simulink model "VAS_LEVEL0_TASK1_TIME"  (Simulink 3.00)
libraries: mathlib x438, logiclib x192, paramlib x18, genlib x3, timelib x1
(part 2 of 2)

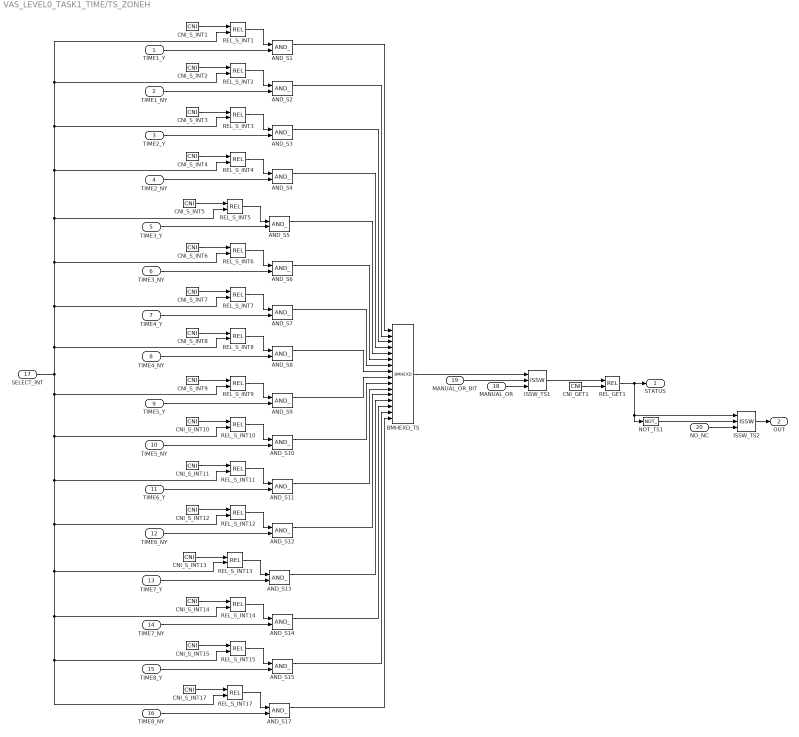
== system VAS_LEVEL0_TASK1_TIME/TS_ZONEH ==
  TIME1_Y : Inport  Port=1
  TIME1_NY : Inport  Port=2
  TIME2_Y : Inport  Port=3
  TIME2_NY : Inport  Port=4
  TIME3_Y : Inport  Port=5
  TIME3_NY : Inport  Port=6
  TIME4_Y : Inport  Port=7
  TIME4_NY : Inport  Port=8
  TIME5_Y : Inport  Port=9
  TIME5_NY : Inport  Port=10
  TIME6_Y : Inport  Port=11
  TIME6_NY : Inport  Port=12
  TIME7_Y : Inport  Port=13
  TIME7_NY : Inport  Port=14
  TIME8_Y : Inport  Port=15
  TIME8_NY : Inport  Port=16
  SELECT_INT : Inport  Port=17
  MANUAL_OR : Inport  Port=18
  MANUAL_OR_BIT : Inport  Port=19
  NO_NC : Inport  Port=20
  AND_S{1..15,17} (16 alike) : logiclib/AND_
  BMHEXD_TS : logiclib/BMHEXD  shift=0
  CNI_GET1 : mathlib/CNI  icn=1
  CNI_S_INT1 : mathlib/CNI  icn=0
  CNI_S_INT10 : mathlib/CNI  icn=9
  CNI_S_INT11 : mathlib/CNI  icn=10
  CNI_S_INT12 : mathlib/CNI  icn=11
  CNI_S_INT13 : mathlib/CNI  icn=12
  CNI_S_INT14 : mathlib/CNI  icn=13
  CNI_S_INT15 : mathlib/CNI  icn=14
  CNI_S_INT17 : mathlib/CNI  icn=15
  CNI_S_INT2 : mathlib/CNI  icn=1
  CNI_S_INT3 : mathlib/CNI  icn=2
  CNI_S_INT4 : mathlib/CNI  icn=3
  CNI_S_INT5 : mathlib/CNI  icn=4
  CNI_S_INT6 : mathlib/CNI  icn=5
  CNI_S_INT7 : mathlib/CNI  icn=6
  CNI_S_INT8 : mathlib/CNI  icn=7
  CNI_S_INT9 : mathlib/CNI  icn=8
  ISSW_TS1 : logiclib/ISSW
  ISSW_TS2 : logiclib/ISSW
  NOT_TS1 : logiclib/NOT_
  REL_GET1 : mathlib/REL  irel=6: greater or equal (>=)
  REL_S_INT{1..15,17} (16 alike) : mathlib/REL  irel=1: equality (==)
  STATUS : Outport  Port=1
  OUT : Outport  Port=2
  wires:
  AND_S1/1 -> BMHEXD_TS/1
  AND_S10/1 -> BMHEXD_TS/10
  AND_S11/1 -> BMHEXD_TS/11
  AND_S12/1 -> BMHEXD_TS/12
  AND_S13/1 -> BMHEXD_TS/13
  AND_S14/1 -> BMHEXD_TS/14
  AND_S15/1 -> BMHEXD_TS/15
  AND_S17/1 -> BMHEXD_TS/16
  AND_S2/1 -> BMHEXD_TS/2
  AND_S3/1 -> BMHEXD_TS/3
  AND_S4/1 -> BMHEXD_TS/4
  AND_S5/1 -> BMHEXD_TS/5
  AND_S6/1 -> BMHEXD_TS/6
  AND_S7/1 -> BMHEXD_TS/7
  AND_S8/1 -> BMHEXD_TS/8
  AND_S9/1 -> BMHEXD_TS/9
  BMHEXD_TS/1 -> ISSW_TS1/1
  CNI_GET1/1 -> REL_GET1/2
  CNI_S_INT1/1 -> REL_S_INT1/1
  CNI_S_INT10/1 -> REL_S_INT10/1
  CNI_S_INT11/1 -> REL_S_INT11/1
  CNI_S_INT12/1 -> REL_S_INT12/1
  CNI_S_INT13/1 -> REL_S_INT13/1
  CNI_S_INT14/1 -> REL_S_INT14/1
  CNI_S_INT15/1 -> REL_S_INT15/1
  CNI_S_INT17/1 -> REL_S_INT17/1
  CNI_S_INT2/1 -> REL_S_INT2/1
  CNI_S_INT3/1 -> REL_S_INT3/1
  CNI_S_INT4/1 -> REL_S_INT4/1
  CNI_S_INT5/1 -> REL_S_INT5/1
  CNI_S_INT6/1 -> REL_S_INT6/1
  CNI_S_INT7/1 -> REL_S_INT7/1
  CNI_S_INT8/1 -> REL_S_INT8/1
  CNI_S_INT9/1 -> REL_S_INT9/1
  ISSW_TS1/1 -> REL_GET1/1
  ISSW_TS2/1 -> OUT/1
  MANUAL_OR/1 -> ISSW_TS1/3
  MANUAL_OR_BIT/1 -> ISSW_TS1/2
  NOT_TS1/1 -> ISSW_TS2/2
  NO_NC/1 -> ISSW_TS2/3
  REL_GET1/1 -> STATUS/1, ISSW_TS2/1, NOT_TS1/1
  REL_S_INT1/1 -> AND_S1/1
  REL_S_INT10/1 -> AND_S10/1
  REL_S_INT11/1 -> AND_S11/1
  REL_S_INT12/1 -> AND_S12/1
  REL_S_INT13/1 -> AND_S13/1
  REL_S_INT14/1 -> AND_S14/1
  REL_S_INT15/1 -> AND_S15/1
  REL_S_INT17/1 -> AND_S17/1
  REL_S_INT2/1 -> AND_S2/1
  REL_S_INT3/1 -> AND_S3/1
  REL_S_INT4/1 -> AND_S4/1
  REL_S_INT5/1 -> AND_S5/1
  REL_S_INT6/1 -> AND_S6/1
  REL_S_INT7/1 -> AND_S7/1
  REL_S_INT8/1 -> AND_S8/1
  REL_S_INT9/1 -> AND_S9/1
  SELECT_INT/1 -> REL_S_INT1/2, REL_S_INT2/2, REL_S_INT3/2, REL_S_INT4/2, REL_S_INT5/2, REL_S_INT6/2, REL_S_INT7/2, REL_S_INT8/2, REL_S_INT14/2, REL_S_INT15/2, REL_S_INT17/2, REL_S_INT13/2, REL_S_INT12/2, REL_S_INT11/2, REL_S_INT10/2, REL_S_INT9/2
  TIME1_NY/1 -> AND_S2/2
  TIME1_Y/1 -> AND_S1/2
  TIME2_NY/1 -> AND_S4/2
  TIME2_Y/1 -> AND_S3/2
  TIME3_NY/1 -> AND_S6/2
  TIME3_Y/1 -> AND_S5/2
  TIME4_NY/1 -> AND_S8/2
  TIME4_Y/1 -> AND_S7/2
  TIME5_NY/1 -> AND_S10/2
  TIME5_Y/1 -> AND_S9/2
  TIME6_NY/1 -> AND_S12/2
  TIME6_Y/1 -> AND_S11/2
  TIME7_NY/1 -> AND_S14/2
  TIME7_Y/1 -> AND_S13/2
  TIME8_NY/1 -> AND_S17/2
  TIME8_Y/1 -> AND_S15/2

== system VAS_LEVEL0_TASK1_TIME/EPHEM_CTBE/EPHEM_BEGIN ==
  ENABLE : Inport  Port=1
  ADD_AMS : mathlib/ADD
  ADD_HM : mathlib/ADD
  CNI_IMUL_H : mathlib/CNI  icn=3600
  CNI_IMUL_M : mathlib/CNI  icn=60
  MUL_H : mathlib/MUL
  MUL_M : mathlib/MUL
  SILO_HOUR : paramlib/SILO  fname=/ramdisk/begin_civil_twilight/loc_hour.txt  CSF=off  CLF=off  yerr=0
  SILO_MINUTE : paramlib/SILO  fname=/ramdisk/begin_civil_twilight/loc_minute.txt  CSF=off  CLF=off  yerr=0
  SILO_SECONDS : paramlib/SILO  fname=/ramdisk/begin_civil_twilight/loc_secound.txt  CSF=off  CLF=off  yerr=0
  HOUR : Outport  Port=1
  MINUTE : Outport  Port=2
  SECONDS : Outport  Port=3
  SEC_OF_DAY : Outport  Port=4
  wires:
  ADD_AMS/1 -> SEC_OF_DAY/1
  ADD_HM/1 -> ADD_AMS/1
  CNI_IMUL_H/1 -> MUL_H/2
  CNI_IMUL_M/1 -> MUL_M/2
  ENABLE/1 -> SILO_HOUR/3, SILO_MINUTE/3, SILO_SECONDS/3
  MUL_H/1 -> ADD_HM/1
  MUL_M/1 -> ADD_HM/2
  SILO_HOUR/1 -> HOUR/1, MUL_H/1
  SILO_MINUTE/1 -> MINUTE/1, MUL_M/1
  SILO_SECONDS/1 -> ADD_AMS/2, SECONDS/1

== system VAS_LEVEL0_TASK1_TIME/EPHEM_CTBE/EPHEM_END ==
  ENABLE : Inport  Port=1
  ADD_AMS : mathlib/ADD
  ADD_HM : mathlib/ADD
  CNI_IMUL_H : mathlib/CNI  icn=3600
  CNI_IMUL_M : mathlib/CNI  icn=60
  MUL_H : mathlib/MUL
  MUL_M : mathlib/MUL
  SILO_HOUR : paramlib/SILO  fname=/ramdisk/end_civil_twilight/loc_hour.txt  CSF=off  CLF=off  yerr=0
  SILO_MINUTE : paramlib/SILO  fname=/ramdisk/end_civil_twilight/loc_minute.txt  CSF=off  CLF=off  yerr=0
  SILO_SECONDS : paramlib/SILO  fname=/ramdisk/end_civil_twilight/loc_second.txt  CSF=off  CLF=off  yerr=0
  HOUR : Outport  Port=1
  MINUTE : Outport  Port=2
  SECONDS : Outport  Port=3
  SEC_OF_DAY : Outport  Port=4
  wires:
  ADD_AMS/1 -> SEC_OF_DAY/1
  ADD_HM/1 -> ADD_AMS/1
  CNI_IMUL_H/1 -> MUL_H/2
  CNI_IMUL_M/1 -> MUL_M/2
  ENABLE/1 -> SILO_HOUR/3, SILO_MINUTE/3, SILO_SECONDS/3
  MUL_H/1 -> ADD_HM/1
  MUL_M/1 -> ADD_HM/2
  SILO_HOUR/1 -> HOUR/1, MUL_H/1
  SILO_MINUTE/1 -> MINUTE/1, MUL_M/1
  SILO_SECONDS/1 -> ADD_AMS/2, SECONDS/1

== system VAS_LEVEL0_TASK1_TIME/EPHEM_MRBE/EPHEM_MRB ==
  ENABLE : Inport  Port=1
  ADD_AMS : mathlib/ADD
  ADD_HM : mathlib/ADD
  CNI_IMUL_H : mathlib/CNI  icn=3600
  CNI_IMUL_M : mathlib/CNI  icn=60
  MUL_H : mathlib/MUL
  MUL_M : mathlib/MUL
  SILO_MR_TIME_H : paramlib/SILO  fname=/ramdisk/moonrise/loc_hour.txt  CSF=off  CLF=off  yerr=0
  SILO_MR_TIME_M : paramlib/SILO  fname=/ramdisk/moonrise/loc_minute.txt  CSF=off  CLF=off  yerr=0
  SILO_MR_TIME_S : paramlib/SILO  fname=/ramdisk/moonrise/loc_second.txt  CSF=off  CLF=off  yerr=0
  MR_HOUR : Outport  Port=1
  MR_MIN : Outport  Port=2
  MR_SEC : Outport  Port=3
  MR_SOD : Outport  Port=4
  wires:
  ADD_AMS/1 -> MR_SOD/1
  ADD_HM/1 -> ADD_AMS/1
  CNI_IMUL_H/1 -> MUL_H/2
  CNI_IMUL_M/1 -> MUL_M/2
  ENABLE/1 -> SILO_MR_TIME_H/3, SILO_MR_TIME_M/3, SILO_MR_TIME_S/3
  MUL_H/1 -> ADD_HM/1
  MUL_M/1 -> ADD_HM/2
  SILO_MR_TIME_H/1 -> MR_HOUR/1, MUL_H/1
  SILO_MR_TIME_M/1 -> MR_MIN/1, MUL_M/1
  SILO_MR_TIME_S/1 -> ADD_AMS/2, MR_SEC/1

== system VAS_LEVEL0_TASK1_TIME/EPHEM_MRBE/EPHEM_MSE ==
  ENABLE : Inport  Port=1
  ADD_AMS : mathlib/ADD
  ADD_HM : mathlib/ADD
  CNI_IMUL_H : mathlib/CNI  icn=3600
  CNI_IMUL_M : mathlib/CNI  icn=60
  MUL_H : mathlib/MUL
  MUL_M : mathlib/MUL
  SILO_MS_TIME_H : paramlib/SILO  fname=/ramdisk/moonset/loc_hour.txt  CSF=off  CLF=off  yerr=0
  SILO_MS_TIME_M : paramlib/SILO  fname=/ramdisk/moonset/loc_minute.txt  CSF=off  CLF=off  yerr=0
  SILO_MS_TIME_S : paramlib/SILO  fname=/ramdisk/moonset/loc_second.txt  CSF=off  CLF=off  yerr=0
  MS_HOUR : Outport  Port=1
  MS_MIN : Outport  Port=2
  MS_SEC : Outport  Port=3
  MS_SOD : Outport  Port=4
  wires:
  ADD_AMS/1 -> MS_SOD/1
  ADD_HM/1 -> ADD_AMS/1
  CNI_IMUL_H/1 -> MUL_H/2
  CNI_IMUL_M/1 -> MUL_M/2
  ENABLE/1 -> SILO_MS_TIME_H/3, SILO_MS_TIME_M/3, SILO_MS_TIME_S/3
  MUL_H/1 -> ADD_HM/1
  MUL_M/1 -> ADD_HM/2
  SILO_MS_TIME_H/1 -> MS_HOUR/1, MUL_H/1
  SILO_MS_TIME_M/1 -> MS_MIN/1, MUL_M/1
  SILO_MS_TIME_S/1 -> ADD_AMS/2, MS_SEC/1

== system VAS_LEVEL0_TASK1_TIME/EPHEM_SRBE/EPHEM_BEGIN ==
  ENABLE : Inport  Port=1
  ADD_AMS : mathlib/ADD
  ADD_HM : mathlib/ADD
  CNI_IMUL_H : mathlib/CNI  icn=3600
  CNI_IMUL_M : mathlib/CNI  icn=60
  MUL_H : mathlib/MUL
  MUL_M : mathlib/MUL
  SILO_HOUR : paramlib/SILO  fname=/ramdisk/sunrise/loc_hour.txt  CSF=off  CLF=off  yerr=0
  SILO_MINUTE : paramlib/SILO  fname=/ramdisk/sunrise/loc_minute.txt  CSF=off  CLF=off  yerr=0
  SILO_SECONDS : paramlib/SILO  fname=/ramdisk/sunrise/loc_second.txt  CSF=off  CLF=off  yerr=0
  HOUR : Outport  Port=1
  MINUTE : Outport  Port=2
  SECONDS : Outport  Port=3
  SEC_OF_DAY : Outport  Port=4
  wires:
  ADD_AMS/1 -> SEC_OF_DAY/1
  ADD_HM/1 -> ADD_AMS/1
  CNI_IMUL_H/1 -> MUL_H/2
  CNI_IMUL_M/1 -> MUL_M/2
  ENABLE/1 -> SILO_HOUR/3, SILO_MINUTE/3, SILO_SECONDS/3
  MUL_H/1 -> ADD_HM/1
  MUL_M/1 -> ADD_HM/2
  SILO_HOUR/1 -> HOUR/1, MUL_H/1
  SILO_MINUTE/1 -> MINUTE/1, MUL_M/1
  SILO_SECONDS/1 -> ADD_AMS/2, SECONDS/1

== system VAS_LEVEL0_TASK1_TIME/EPHEM_SRBE/EPHEM_END ==
  ENABLE : Inport  Port=1
  ADD_AMS : mathlib/ADD
  ADD_HM : mathlib/ADD
  CNI_IMUL_H : mathlib/CNI  icn=3600
  CNI_IMUL_M : mathlib/CNI  icn=60
  MUL_H : mathlib/MUL
  MUL_M : mathlib/MUL
  SILO_HOUR : paramlib/SILO  fname=/ramdisk/sunset/loc_hour.txt  CSF=off  CLF=off  yerr=0
  SILO_MINUTE : paramlib/SILO  fname=/ramdisk/sunset/loc_minute.txt  CSF=off  CLF=off  yerr=0
  SILO_SECONDS : paramlib/SILO  fname=/ramdisk/sunset/loc_second.txt  CSF=off  CLF=off  yerr=0
  HOUR : Outport  Port=1
  MINUTE : Outport  Port=2
  SECONDS : Outport  Port=3
  SEC_OF_DAY : Outport  Port=4
  wires:
  ADD_AMS/1 -> SEC_OF_DAY/1
  ADD_HM/1 -> ADD_AMS/1
  CNI_IMUL_H/1 -> MUL_H/2
  CNI_IMUL_M/1 -> MUL_M/2
  ENABLE/1 -> SILO_HOUR/3, SILO_MINUTE/3, SILO_SECONDS/3
  MUL_H/1 -> ADD_HM/1
  MUL_M/1 -> ADD_HM/2
  SILO_HOUR/1 -> HOUR/1, MUL_H/1
  SILO_MINUTE/1 -> MINUTE/1, MUL_M/1
  SILO_SECONDS/1 -> ADD_AMS/2, SECONDS/1

== system VAS_LEVEL0_TASK1_TIME/MANUAL_BE0/MANUAL_BEGIN ==
  IN_HOUR : Inport  Port=1
  IN_MINUTE : Inport  Port=2
  IN_SECONDS : Inport  Port=3
  ADD_AMS : mathlib/ADD
  ADD_HM : mathlib/ADD
  CNI_IMUL_H : mathlib/CNI  icn=3600
  CNI_IMUL_M : mathlib/CNI  icn=60
  MUL_H : mathlib/MUL
  MUL_M : mathlib/MUL
  HOUR : Outport  Port=1
  MINUTE : Outport  Port=2
  SECONDS : Outport  Port=3
  SEC_OF_DAY : Outport  Port=4
  wires:
  ADD_AMS/1 -> SEC_OF_DAY/1
  ADD_HM/1 -> ADD_AMS/1
  CNI_IMUL_H/1 -> MUL_H/2
  CNI_IMUL_M/1 -> MUL_M/2
  IN_HOUR/1 -> HOUR/1, MUL_H/1
  IN_MINUTE/1 -> MINUTE/1, MUL_M/1
  IN_SECONDS/1 -> ADD_AMS/2, SECONDS/1
  MUL_H/1 -> ADD_HM/1
  MUL_M/1 -> ADD_HM/2

== system VAS_LEVEL0_TASK1_TIME/MANUAL_BE0/MANUAL_END ==
  IN_HOUR : Inport  Port=1
  IN_MINUTE : Inport  Port=2
  IN_SECONDS : Inport  Port=3
  ADD_AMS : mathlib/ADD
  ADD_HM : mathlib/ADD
  CNI_IMUL_H : mathlib/CNI  icn=3600
  CNI_IMUL_M : mathlib/CNI  icn=60
  MUL_H : mathlib/MUL
  MUL_M : mathlib/MUL
  HOUR : Outport  Port=1
  MINUTE : Outport  Port=2
  SECONDS : Outport  Port=3
  SEC_OF_DAY : Outport  Port=4
  wires:
  ADD_AMS/1 -> SEC_OF_DAY/1
  ADD_HM/1 -> ADD_AMS/1
  CNI_IMUL_H/1 -> MUL_H/2
  CNI_IMUL_M/1 -> MUL_M/2
  IN_HOUR/1 -> HOUR/1, MUL_H/1
  IN_MINUTE/1 -> MINUTE/1, MUL_M/1
  IN_SECONDS/1 -> ADD_AMS/2, SECONDS/1
  MUL_H/1 -> ADD_HM/1
  MUL_M/1 -> ADD_HM/2

== system VAS_LEVEL0_TASK1_TIME/MANUAL_BE1/MANUAL_BEGIN ==
  IN_HOUR : Inport  Port=1
  IN_MINUTE : Inport  Port=2
  IN_SECONDS : Inport  Port=3
  ADD_AMS : mathlib/ADD
  ADD_HM : mathlib/ADD
  CNI_IMUL_H : mathlib/CNI  icn=3600
  CNI_IMUL_M : mathlib/CNI  icn=60
  MUL_H : mathlib/MUL
  MUL_M : mathlib/MUL
  HOUR : Outport  Port=1
  MINUTE : Outport  Port=2
  SECONDS : Outport  Port=3
  SEC_OF_DAY : Outport  Port=4
  wires:
  ADD_AMS/1 -> SEC_OF_DAY/1
  ADD_HM/1 -> ADD_AMS/1
  CNI_IMUL_H/1 -> MUL_H/2
  CNI_IMUL_M/1 -> MUL_M/2
  IN_HOUR/1 -> HOUR/1, MUL_H/1
  IN_MINUTE/1 -> MINUTE/1, MUL_M/1
  IN_SECONDS/1 -> ADD_AMS/2, SECONDS/1
  MUL_H/1 -> ADD_HM/1
  MUL_M/1 -> ADD_HM/2

== system VAS_LEVEL0_TASK1_TIME/MANUAL_BE1/MANUAL_END ==
  IN_HOUR : Inport  Port=1
  IN_MINUTE : Inport  Port=2
  IN_SECONDS : Inport  Port=3
  ADD_AMS : mathlib/ADD
  ADD_HM : mathlib/ADD
  CNI_IMUL_H : mathlib/CNI  icn=3600
  CNI_IMUL_M : mathlib/CNI  icn=60
  MUL_H : mathlib/MUL
  MUL_M : mathlib/MUL
  HOUR : Outport  Port=1
  MINUTE : Outport  Port=2
  SECONDS : Outport  Port=3
  SEC_OF_DAY : Outport  Port=4
  wires:
  ADD_AMS/1 -> SEC_OF_DAY/1
  ADD_HM/1 -> ADD_AMS/1
  CNI_IMUL_H/1 -> MUL_H/2
  CNI_IMUL_M/1 -> MUL_M/2
  IN_HOUR/1 -> HOUR/1, MUL_H/1
  IN_MINUTE/1 -> MINUTE/1, MUL_M/1
  IN_SECONDS/1 -> ADD_AMS/2, SECONDS/1
  MUL_H/1 -> ADD_HM/1
  MUL_M/1 -> ADD_HM/2

== system VAS_LEVEL0_TASK1_TIME/MANUAL_BE2/MANUAL_BEGIN ==
  IN_HOUR : Inport  Port=1
  IN_MINUTE : Inport  Port=2
  IN_SECONDS : Inport  Port=3
  ADD_AMS : mathlib/ADD
  ADD_HM : mathlib/ADD
  CNI_IMUL_H : mathlib/CNI  icn=3600
  CNI_IMUL_M : mathlib/CNI  icn=60
  MUL_H : mathlib/MUL
  MUL_M : mathlib/MUL
  HOUR : Outport  Port=1
  MINUTE : Outport  Port=2
  SECONDS : Outport  Port=3
  SEC_OF_DAY : Outport  Port=4
  wires:
  ADD_AMS/1 -> SEC_OF_DAY/1
  ADD_HM/1 -> ADD_AMS/1
  CNI_IMUL_H/1 -> MUL_H/2
  CNI_IMUL_M/1 -> MUL_M/2
  IN_HOUR/1 -> HOUR/1, MUL_H/1
  IN_MINUTE/1 -> MINUTE/1, MUL_M/1
  IN_SECONDS/1 -> ADD_AMS/2, SECONDS/1
  MUL_H/1 -> ADD_HM/1
  MUL_M/1 -> ADD_HM/2

== system VAS_LEVEL0_TASK1_TIME/MANUAL_BE2/MANUAL_END ==
  IN_HOUR : Inport  Port=1
  IN_MINUTE : Inport  Port=2
  IN_SECONDS : Inport  Port=3
  ADD_AMS : mathlib/ADD
  ADD_HM : mathlib/ADD
  CNI_IMUL_H : mathlib/CNI  icn=3600
  CNI_IMUL_M : mathlib/CNI  icn=60
  MUL_H : mathlib/MUL
  MUL_M : mathlib/MUL
  HOUR : Outport  Port=1
  MINUTE : Outport  Port=2
  SECONDS : Outport  Port=3
  SEC_OF_DAY : Outport  Port=4
  wires:
  ADD_AMS/1 -> SEC_OF_DAY/1
  ADD_HM/1 -> ADD_AMS/1
  CNI_IMUL_H/1 -> MUL_H/2
  CNI_IMUL_M/1 -> MUL_M/2
  IN_HOUR/1 -> HOUR/1, MUL_H/1
  IN_MINUTE/1 -> MINUTE/1, MUL_M/1
  IN_SECONDS/1 -> ADD_AMS/2, SECONDS/1
  MUL_H/1 -> ADD_HM/1
  MUL_M/1 -> ADD_HM/2

== system VAS_LEVEL0_TASK1_TIME/MANUAL_BE3/MANUAL_BEGIN ==
  IN_HOUR : Inport  Port=1
  IN_MINUTE : Inport  Port=2
  IN_SECONDS : Inport  Port=3
  ADD_AMS : mathlib/ADD
  ADD_HM : mathlib/ADD
  CNI_IMUL_H : mathlib/CNI  icn=3600
  CNI_IMUL_M : mathlib/CNI  icn=60
  MUL_H : mathlib/MUL
  MUL_M : mathlib/MUL
  HOUR : Outport  Port=1
  MINUTE : Outport  Port=2
  SECONDS : Outport  Port=3
  SEC_OF_DAY : Outport  Port=4
  wires:
  ADD_AMS/1 -> SEC_OF_DAY/1
  ADD_HM/1 -> ADD_AMS/1
  CNI_IMUL_H/1 -> MUL_H/2
  CNI_IMUL_M/1 -> MUL_M/2
  IN_HOUR/1 -> HOUR/1, MUL_H/1
  IN_MINUTE/1 -> MINUTE/1, MUL_M/1
  IN_SECONDS/1 -> ADD_AMS/2, SECONDS/1
  MUL_H/1 -> ADD_HM/1
  MUL_M/1 -> ADD_HM/2

== system VAS_LEVEL0_TASK1_TIME/MANUAL_BE3/MANUAL_END ==
  IN_HOUR : Inport  Port=1
  IN_MINUTE : Inport  Port=2
  IN_SECONDS : Inport  Port=3
  ADD_AMS : mathlib/ADD
  ADD_HM : mathlib/ADD
  CNI_IMUL_H : mathlib/CNI  icn=3600
  CNI_IMUL_M : mathlib/CNI  icn=60
  MUL_H : mathlib/MUL
  MUL_M : mathlib/MUL
  HOUR : Outport  Port=1
  MINUTE : Outport  Port=2
  SECONDS : Outport  Port=3
  SEC_OF_DAY : Outport  Port=4
  wires:
  ADD_AMS/1 -> SEC_OF_DAY/1
  ADD_HM/1 -> ADD_AMS/1
  CNI_IMUL_H/1 -> MUL_H/2
  CNI_IMUL_M/1 -> MUL_M/2
  IN_HOUR/1 -> HOUR/1, MUL_H/1
  IN_MINUTE/1 -> MINUTE/1, MUL_M/1
  IN_SECONDS/1 -> ADD_AMS/2, SECONDS/1
  MUL_H/1 -> ADD_HM/1
  MUL_M/1 -> ADD_HM/2

== system VAS_LEVEL0_TASK1_TIME/MANUAL_BE4/MANUAL_BEGIN ==
  IN_HOUR : Inport  Port=1
  IN_MINUTE : Inport  Port=2
  IN_SECONDS : Inport  Port=3
  ADD_AMS : mathlib/ADD
  ADD_HM : mathlib/ADD
  CNI_IMUL_H : mathlib/CNI  icn=3600
  CNI_IMUL_M : mathlib/CNI  icn=60
  MUL_H : mathlib/MUL
  MUL_M : mathlib/MUL
  HOUR : Outport  Port=1
  MINUTE : Outport  Port=2
  SECONDS : Outport  Port=3
  SEC_OF_DAY : Outport  Port=4
  wires:
  ADD_AMS/1 -> SEC_OF_DAY/1
  ADD_HM/1 -> ADD_AMS/1
  CNI_IMUL_H/1 -> MUL_H/2
  CNI_IMUL_M/1 -> MUL_M/2
  IN_HOUR/1 -> HOUR/1, MUL_H/1
  IN_MINUTE/1 -> MINUTE/1, MUL_M/1
  IN_SECONDS/1 -> ADD_AMS/2, SECONDS/1
  MUL_H/1 -> ADD_HM/1
  MUL_M/1 -> ADD_HM/2

== system VAS_LEVEL0_TASK1_TIME/MANUAL_BE4/MANUAL_END ==
  IN_HOUR : Inport  Port=1
  IN_MINUTE : Inport  Port=2
  IN_SECONDS : Inport  Port=3
  ADD_AMS : mathlib/ADD
  ADD_HM : mathlib/ADD
  CNI_IMUL_H : mathlib/CNI  icn=3600
  CNI_IMUL_M : mathlib/CNI  icn=60
  MUL_H : mathlib/MUL
  MUL_M : mathlib/MUL
  HOUR : Outport  Port=1
  MINUTE : Outport  Port=2
  SECONDS : Outport  Port=3
  SEC_OF_DAY : Outport  Port=4
  wires:
  ADD_AMS/1 -> SEC_OF_DAY/1
  ADD_HM/1 -> ADD_AMS/1
  CNI_IMUL_H/1 -> MUL_H/2
  CNI_IMUL_M/1 -> MUL_M/2
  IN_HOUR/1 -> HOUR/1, MUL_H/1
  IN_MINUTE/1 -> MINUTE/1, MUL_M/1
  IN_SECONDS/1 -> ADD_AMS/2, SECONDS/1
  MUL_H/1 -> ADD_HM/1
  MUL_M/1 -> ADD_HM/2
